simulink model "animation"  (R2018b)
settings: Solver=VariableStepAuto  StartTime=0.0  StopTime=281.0754  FixedStep=0.01  RelTol=1e-3  EnableMultiTasking=on
values from neighbouring files (symbols this model uses):
  cm = [[0.3;49.6;82],[355.2;24;0.7],[9.8;0;36.7],[0.1;246;20],[0;13.9;55],[0;0;59]]    [dynamics.m]    (also in invDynController.m)
  D = generalizedInertiaMatrix(q,rho,DH,m,cm,I)    [dynamics.m]    (also in generalizedInertiaMatrix.m = D + (Si*J(:,:,i))'*Mc_i*(Si*J(:,:,i)); invDynController.m; motionPlanning.m = size(q_new,2); trajGen.m = size(q,1))
  m = [9 4.3 1.9 1.7 0.3 0.1]    [dynamics.m]    (also in invDynController.m)
  N = numel(pos_list)    [missionPlanning.m]    (also in motionPlanning.m = size(q_new,1); simManipulator.m = numel(Path(:,1)); trajGen.m = size(q,2); trajGen_fmincon.m = size(q,2))
undefined symbols (not defined in the file or in its folder): X, Y, Z
libraries: sm_lib x142, nesl_utility x51, simulink x2
(part 2 of 4)

== system animation/Plant/Link5 ==
  Reference Frame4 : sm_lib/Frames and Transforms/Reference Frame
  Revolute Joint4 : sm_lib/Joints/Revolute Joint  SenseConstraintForce=off  SenseConstraintForceX=off  SenseConstraintForceY=off  SenseConstraintForceZ=off  SenseConstraintTorque=off  SenseConstraintTorqueX=off  SenseConstraintTorqueY=off  SenseConstraintTorqueZ=off  SenseTotalForce=off  SenseTotalForceX=off  SenseTotalForceY=off  SenseTotalForceZ=off  SenseTotalTorque=off  SenseTotalTorqueX=off  SenseTotalTorqueY=off  SenseTotalTorqueZ=off  CompositeWrenchDir=FollowerOnBase  CompositeWrenchFrame=BaseFrame  EquilibriumPosition=0  EquilibriumPositionUnits=deg  SpringStiffness=0  SpringStiffnessUnits=N*m/deg  DampingCoefficient=0  DampingCoefficientUnits=N*m/(deg/s)  TorqueActuationMode=InputTorque  MotionActuationMode=ComputedMotion  SensePosition=on  SenseVelocity=on  SenseAcceleration=off  SenseTorqueForce=on  PositionTargetSpecify=on  PositionTargetPriority=High  PositionTargetValue=0  PositionTargetValueUnits=deg  VelocityTargetSpecify=on  VelocityTargetPriority=High  VelocityTargetValue=0  VelocityTargetValueUnits=deg/s
  Rigid Transform13 : sm_lib/Frames and Transforms/Rigid Transform  TranslationMethod=None  TranslationStandardOffset=0  TranslationLengthUnit=m  TranslationStandardAxis=+Z  TranslationCartesianOffset=[0 0 0]  TranslationROffset=0  TranslationROffsetUnits=m  TranslationZOffset=0  TranslationZOffsetUnits=m  TranslationThetaOffset=0  TranslationThetaOffsetUnits=deg  RotationMethod=StandardAxis  RotationAngleUnits=rad  RotationStandardAxis=+Z  RotationAngle=-pi/6  RotationArbitraryAxis=[0 0 1]  FollAlignAxisA=+X  BaseAlignAxisA=+Y  FollAlignAxisB=+Y  BaseAlignAxisB=+Z  RotationSequenceAxes=FollowerAxes  RotationSequence=XYX  RotationSequenceAngles=[0 0 0]  RotationSequenceAnglesUnits=deg  RotationMatrix=[1 0 0; 0 1 0; 0 0 1]
  Rigid Transform14 : sm_lib/Frames and Transforms/Rigid Transform  TranslationMethod=None  TranslationStandardOffset=250.5  TranslationLengthUnit=mm  TranslationStandardAxis=+Z  TranslationCartesianOffset=[0 0 0]  TranslationROffset=0  TranslationROffsetUnits=m  TranslationZOffset=0  TranslationZOffsetUnits=m  TranslationThetaOffset=0  TranslationThetaOffsetUnits=deg  RotationMethod=None  RotationAngleUnits=deg  RotationStandardAxis=+Z  RotationAngle=0.0  RotationArbitraryAxis=[0 0 1]  FollAlignAxisA=+X  BaseAlignAxisA=+Y  FollAlignAxisB=+Y  BaseAlignAxisB=+Z  RotationSequenceAxes=FollowerAxes  RotationSequence=XYX  RotationSequenceAngles=[0 0 0]  RotationSequenceAnglesUnits=deg  RotationMatrix=[1 0 0; 0 1 0; 0 0 1]
  Rigid Transform15 : sm_lib/Frames and Transforms/Rigid Transform  TranslationMethod=None  TranslationStandardOffset=0  TranslationLengthUnit=m  TranslationStandardAxis=+Z  TranslationCartesianOffset=[0 0 0]  TranslationROffset=0  TranslationROffsetUnits=m  TranslationZOffset=0  TranslationZOffsetUnits=m  TranslationThetaOffset=0  TranslationThetaOffsetUnits=deg  RotationMethod=None  RotationAngleUnits=rad  RotationStandardAxis=+X  RotationAngle=pi/2  RotationArbitraryAxis=[0 0 1]  FollAlignAxisA=+X  BaseAlignAxisA=+Y  FollAlignAxisB=+Y  BaseAlignAxisB=+Z  RotationSequenceAxes=FollowerAxes  RotationSequence=XYX  RotationSequenceAngles=[0 0 0]  RotationSequenceAnglesUnits=deg  RotationMatrix=[1 0 0; 0 1 0; 0 0 1]
  Rigid Transform20 : sm_lib/Frames and Transforms/Rigid Transform  TranslationMethod=None  TranslationStandardOffset=500  TranslationLengthUnit=mm  TranslationStandardAxis=+X  TranslationCartesianOffset=[0 0 0]  TranslationROffset=0  TranslationROffsetUnits=m  TranslationZOffset=0  TranslationZOffsetUnits=m  TranslationThetaOffset=0  TranslationThetaOffsetUnits=deg  RotationMethod=StandardAxis  RotationAngleUnits=rad  RotationStandardAxis=+X  RotationAngle=-pi/2  RotationArbitraryAxis=[0 0 1]  FollAlignAxisA=+X  BaseAlignAxisA=+Y  FollAlignAxisB=+Y  BaseAlignAxisB=+Z  RotationSequenceAxes=FollowerAxes  RotationSequence=XYX  RotationSequenceAngles=[0 0 0]  RotationSequenceAnglesUnits=deg  RotationMatrix=[1 0 0; 0 1 0; 0 0 1]
  Solid5 : sm_lib/Body Elements/Solid  InertiaType=Custom  Mass=0.87  MassUnits=kg  CenterOfMass=[0 4.29 -58.96]  CenterOfMassUnits=mm  MomentsOfInertia=[0 0 0]  MomentsOfInertiaUnits=kg*m^2  ProductsOfInertia=[0 0 0]  ProductsOfInertiaUnits=kg*m^2  BasedOnType=Density  Density=1000  DensityUnits=kg/m^3  DoExposeReferenceFrame=on  SerializedFrames=<Frames/>  GraphicType=FromGeometry  MarkerShape=Sphere  MarkerSize=10  GraphicVisPropType=SimpleVisualProperties  GraphicDiffuseColor=[1.0 1.0 0.0]  GraphicSpecularColor=[0.5 0.5 0.5 1.0]  GraphicAmbientColor=[0.15 0.15 0.15 1.0]  GraphicEmissiveColor=[0.0 0.0 0.0 1.0]  GraphicShininess=75  GraphicOpacity=1.0  GeometryShape=FromFile  RectangleSize=[1 1]  RectangleSizeUnits=m  BrickDimensions=[1 1 1]  BrickDimensionUnits=m  CylinderRadius=1  CylinderRadiusUnits=m  CylinderLength=1  CylinderLengthUnits=m  SphereRadius=1  SphereRadiusUnits=m  EllipsoidRadii=[1 1 1]  EllipsoidRadiiUnits=m  ExtrusionCrossSection=[1 1; -1 1; -1 -1; 1 -1]  ExtrusionCrossSectionUnits=m  ExtrusionLength=1  ExtrusionLengthUnits=m  PolygonNumSides=3  PolygonOuterRadius=1  PolygonOuterRadiusUnits=m  ExtGeomFileType=STL  ExtGeomFileName=D:\Chin\3rdYearsProject\IntroRobotics\Project\CAD\SubAssem6.STL  ExtGeomFileUnits=mm  RevolutionCrossSection=[1 1; 1 -1; 2 -1; 2 1]  RevolutionCrossSectionUnits=m  RevolutionExtent=Full  RevolutionAngle=180  RevolutionAngleUnits=deg
  Frame4 : PMIOPort  Side=Left
  t : PMIOPort  Port=2  Side=Left
  Frame5 : PMIOPort  Port=3  Side=Right
  q : PMIOPort  Port=4  Side=Right
  w : PMIOPort  Port=5  Side=Right
  t_out : PMIOPort  Port=6  Side=Right
  connections:
  Rigid Transform20/RConn1 -- Frame5/RConn1 -- Reference Frame4/RConn1 -- Solid5/RConn1
  Rigid Transform15/LConn1 -- Rigid Transform14/RConn1
  Rigid Transform15/RConn1 -- Rigid Transform20/LConn1
  Rigid Transform13/LConn1 -- Revolute Joint4/RConn1
  Rigid Transform14/LConn1 -- Rigid Transform13/RConn1
  Revolute Joint4/LConn1 -- Frame4/RConn1
  Revolute Joint4/LConn2 -- t/RConn1
  Revolute Joint4/RConn3 -- w/RConn1
  Revolute Joint4/RConn2 -- q/RConn1
  Revolute Joint4/RConn4 -- t_out/RConn1

== system animation/Plant/Link6 ==
  Reference Frame5 : sm_lib/Frames and Transforms/Reference Frame
  Revolute Joint5 : sm_lib/Joints/Revolute Joint  SenseConstraintForce=off  SenseConstraintForceX=off  SenseConstraintForceY=off  SenseConstraintForceZ=off  SenseConstraintTorque=off  SenseConstraintTorqueX=off  SenseConstraintTorqueY=off  SenseConstraintTorqueZ=off  SenseTotalForce=off  SenseTotalForceX=off  SenseTotalForceY=off  SenseTotalForceZ=off  SenseTotalTorque=off  SenseTotalTorqueX=off  SenseTotalTorqueY=off  SenseTotalTorqueZ=off  CompositeWrenchDir=FollowerOnBase  CompositeWrenchFrame=BaseFrame  EquilibriumPosition=0  EquilibriumPositionUnits=deg  SpringStiffness=0  SpringStiffnessUnits=N*m/deg  DampingCoefficient=0  DampingCoefficientUnits=N*m/(deg/s)  TorqueActuationMode=InputTorque  MotionActuationMode=ComputedMotion  SensePosition=on  SenseVelocity=on  SenseAcceleration=off  SenseTorqueForce=on  PositionTargetSpecify=on  PositionTargetPriority=High  PositionTargetValue=0  PositionTargetValueUnits=deg  VelocityTargetSpecify=on  VelocityTargetPriority=High  VelocityTargetValue=0  VelocityTargetValueUnits=deg/s
  Rigid Transform21 : sm_lib/Frames and Transforms/Rigid Transform  TranslationMethod=None  TranslationStandardOffset=0  TranslationLengthUnit=m  TranslationStandardAxis=+Z  TranslationCartesianOffset=[0 0 0]  TranslationROffset=0  TranslationROffsetUnits=m  TranslationZOffset=0  TranslationZOffsetUnits=m  TranslationThetaOffset=0  TranslationThetaOffsetUnits=deg  RotationMethod=None  RotationAngleUnits=rad  RotationStandardAxis=+Z  RotationAngle=-pi/6  RotationArbitraryAxis=[0 0 1]  FollAlignAxisA=+X  BaseAlignAxisA=+Y  FollAlignAxisB=+Y  BaseAlignAxisB=+Z  RotationSequenceAxes=FollowerAxes  RotationSequence=XYX  RotationSequenceAngles=[0 0 0]  RotationSequenceAnglesUnits=deg  RotationMatrix=[1 0 0; 0 1 0; 0 0 1]
  Rigid Transform22 : sm_lib/Frames and Transforms/Rigid Transform  TranslationMethod=StandardAxis  TranslationStandardOffset=230  TranslationLengthUnit=mm  TranslationStandardAxis=-Z  TranslationCartesianOffset=[0 0 0]  TranslationROffset=0  TranslationROffsetUnits=m  TranslationZOffset=0  TranslationZOffsetUnits=m  TranslationThetaOffset=0  TranslationThetaOffsetUnits=deg  RotationMethod=None  RotationAngleUnits=deg  RotationStandardAxis=+Z  RotationAngle=0.0  RotationArbitraryAxis=[0 0 1]  FollAlignAxisA=+X  BaseAlignAxisA=+Y  FollAlignAxisB=+Y  BaseAlignAxisB=+Z  RotationSequenceAxes=FollowerAxes  RotationSequence=XYX  RotationSequenceAngles=[0 0 0]  RotationSequenceAnglesUnits=deg  RotationMatrix=[1 0 0; 0 1 0; 0 0 1]
  Rigid Transform23 : sm_lib/Frames and Transforms/Rigid Transform  TranslationMethod=None  TranslationStandardOffset=0  TranslationLengthUnit=m  TranslationStandardAxis=+Z  TranslationCartesianOffset=[0 0 0]  TranslationROffset=0  TranslationROffsetUnits=m  TranslationZOffset=0  TranslationZOffsetUnits=m  TranslationThetaOffset=0  TranslationThetaOffsetUnits=deg  RotationMethod=None  RotationAngleUnits=rad  RotationStandardAxis=+X  RotationAngle=pi/2  RotationArbitraryAxis=[0 0 1]  FollAlignAxisA=+X  BaseAlignAxisA=+Y  FollAlignAxisB=+Y  BaseAlignAxisB=+Z  RotationSequenceAxes=FollowerAxes  RotationSequence=XYX  RotationSequenceAngles=[0 0 0]  RotationSequenceAnglesUnits=deg  RotationMatrix=[1 0 0; 0 1 0; 0 0 1]
  Rigid Transform24 : sm_lib/Frames and Transforms/Rigid Transform  TranslationMethod=None  TranslationStandardOffset=500  TranslationLengthUnit=mm  TranslationStandardAxis=+X  TranslationCartesianOffset=[0 0 0]  TranslationROffset=0  TranslationROffsetUnits=m  TranslationZOffset=0  TranslationZOffsetUnits=m  TranslationThetaOffset=0  TranslationThetaOffsetUnits=deg  RotationMethod=StandardAxis  RotationAngleUnits=rad  RotationStandardAxis=+X  RotationAngle=pi  RotationArbitraryAxis=[0 0 1]  FollAlignAxisA=+X  BaseAlignAxisA=+Y  FollAlignAxisB=+Y  BaseAlignAxisB=+Z  RotationSequenceAxes=FollowerAxes  RotationSequence=XYX  RotationSequenceAngles=[0 0 0]  RotationSequenceAnglesUnits=deg  RotationMatrix=[1 0 0; 0 1 0; 0 0 1]
  Solid6 : sm_lib/Body Elements/Solid  InertiaType=Custom  Mass=0.115  MassUnits=kg  CenterOfMass=[-1.12 -0.51 -58.13]  CenterOfMassUnits=mm  MomentsOfInertia=[5029.75 5041.84 923.6]  MomentsOfInertiaUnits=g*cm^2  ProductsOfInertia=[39.56 88.09 6.8]  ProductsOfInertiaUnits=g*cm^2  BasedOnType=Density  Density=1000  DensityUnits=kg/m^3  DoExposeReferenceFrame=on  SerializedFrames=<Frames/>  GraphicType=FromGeometry  MarkerShape=Sphere  MarkerSize=10  GraphicVisPropType=SimpleVisualProperties  GraphicDiffuseColor=[0.0 1.0 0.2]  GraphicSpecularColor=[0.5 0.5 0.5 1.0]  GraphicAmbientColor=[0.15 0.15 0.15 1.0]  GraphicEmissiveColor=[0.0 0.0 0.0 1.0]  GraphicShininess=75  GraphicOpacity=1.0  GeometryShape=FromFile  RectangleSize=[1 1]  RectangleSizeUnits=m  BrickDimensions=[1 1 1]  BrickDimensionUnits=m  CylinderRadius=1  CylinderRadiusUnits=m  CylinderLength=1  CylinderLengthUnits=m  SphereRadius=1  SphereRadiusUnits=m  EllipsoidRadii=[1 1 1]  EllipsoidRadiiUnits=m  ExtrusionCrossSection=[1 1; -1 1; -1 -1; 1 -1]  ExtrusionCrossSectionUnits=m  ExtrusionLength=1  ExtrusionLengthUnits=m  PolygonNumSides=3  PolygonOuterRadius=1  PolygonOuterRadiusUnits=m  ExtGeomFileType=STL  ExtGeomFileName=D:\Chin\3rdYearsProject\IntroRobotics\Project\CAD\SubAssem_end_plate2.STL  ExtGeomFileUnits=mm  RevolutionCrossSection=[1 1; 1 -1; 2 -1; 2 1]  RevolutionCrossSectionUnits=m  RevolutionExtent=Full  RevolutionAngle=180  RevolutionAngleUnits=deg
  Frame6 : PMIOPort  Side=Left
  Frame5 : PMIOPort  Port=2  Side=Right
  t : PMIOPort  Port=3  Side=Left
  q : PMIOPort  Port=4  Side=Right
  w : PMIOPort  Port=5  Side=Right
  t_out : PMIOPort  Port=6  Side=Right
  connections:
  Revolute Joint5/LConn2 -- t/RConn1
  Revolute Joint5/RConn3 -- w/RConn1
  Revolute Joint5/RConn2 -- q/RConn1
  Rigid Transform24/RConn1 -- Solid6/RConn1 -- Frame6/RConn1 -- Reference Frame5/RConn1
  Rigid Transform22/LConn1 -- Rigid Transform21/RConn1
  Rigid Transform23/RConn1 -- Rigid Transform24/LConn1
  Rigid Transform23/LConn1 -- Rigid Transform22/RConn1
  Rigid Transform21/LConn1 -- Revolute Joint5/RConn1
  Revolute Joint5/LConn1 -- Frame5/RConn1
  t_out/RConn1 -- Revolute Joint5/RConn4

== system animation/Trajectory Generator/Trajectory1 ==
  t : Inport
  A : Subsystem
  Product : Product  Multiplication=Matrix(*)
  Product1 : Product  Multiplication=Matrix(*)
  Product2 : Product  Multiplication=Matrix(*)
  coef_q : Subsystem
  coef_qd : Subsystem
  coef_qdd : Subsystem
  q_r : Outport
  qd_r : Outport  Port=2
  qdd_r : Outport  Port=3
  wires:
  Product/1 -> q_r/1
  A/1(A) -> Product2/2, Product1/2, Product/2
  coef_qd/1(coef_qd) -> Product1/1
  coef_qdd/1(coef_qdd) -> Product2/1
  t/1 -> coef_qdd/1(t), coef_qd/1(t), coef_q/1(t)
  Product1/1 -> qd_r/1
  coef_q/1(coef_q) -> Product/1
  Product2/1 -> qdd_r/1

== system animation/Trajectory Generator/Trajectory2 ==
  t : Inport
  A : Subsystem
  Product : Product  Multiplication=Matrix(*)
  Product1 : Product  Multiplication=Matrix(*)
  Product2 : Product  Multiplication=Matrix(*)
  coef_q : Subsystem
  coef_qd : Subsystem
  coef_qdd : Subsystem
  q_r : Outport
  qd_r : Outport  Port=2
  qdd_r : Outport  Port=3
  wires:
  Product2/1 -> qdd_r/1
  coef_q/1(coef_q) -> Product/1
  Product1/1 -> qd_r/1
  t/1 -> coef_q/1(t), coef_qd/1(t), coef_qdd/1(t)
  coef_qdd/1(coef_qdd) -> Product2/1
  coef_qd/1(coef_qd) -> Product1/1
  A/1(A) -> Product/2, Product1/2, Product2/2
  Product/1 -> q_r/1

== system animation/Trajectory Generator/Trajectory3 ==
  t : Inport
  A : Subsystem
  Product : Product  Multiplication=Matrix(*)
  Product1 : Product  Multiplication=Matrix(*)
  Product2 : Product  Multiplication=Matrix(*)
  coef_q : Subsystem
  coef_qd : Subsystem
  coef_qdd : Subsystem
  q_r : Outport
  qd_r : Outport  Port=2
  qdd_r : Outport  Port=3
  wires:
  Product/1 -> q_r/1
  A/1(A) -> Product2/2, Product1/2, Product/2
  coef_qd/1(coef_qd) -> Product1/1
  coef_qdd/1(coef_qdd) -> Product2/1
  t/1 -> coef_qdd/1(t), coef_qd/1(t), coef_q/1(t)
  Product1/1 -> qd_r/1
  coef_q/1(coef_q) -> Product/1
  Product2/1 -> qdd_r/1

== system animation/Trajectory Generator1/Trajectory2 ==
  t : Inport
  A : Subsystem
  Product : Product  Multiplication=Matrix(*)
  Product1 : Product  Multiplication=Matrix(*)
  Product2 : Product  Multiplication=Matrix(*)
  coef_q : Subsystem
  coef_qd : Subsystem
  coef_qdd : Subsystem
  q_r : Outport
  qd_r : Outport  Port=2
  qdd_r : Outport  Port=3
  wires:
  Product/1 -> q_r/1
  A/1(A) -> Product2/2, Product1/2, Product/2
  coef_qd/1(coef_qd) -> Product1/1
  coef_qdd/1(coef_qdd) -> Product2/1
  t/1 -> coef_qdd/1(t), coef_qd/1(t), coef_q/1(t)
  Product1/1 -> qd_r/1
  coef_q/1(coef_q) -> Product/1
  Product2/1 -> qdd_r/1

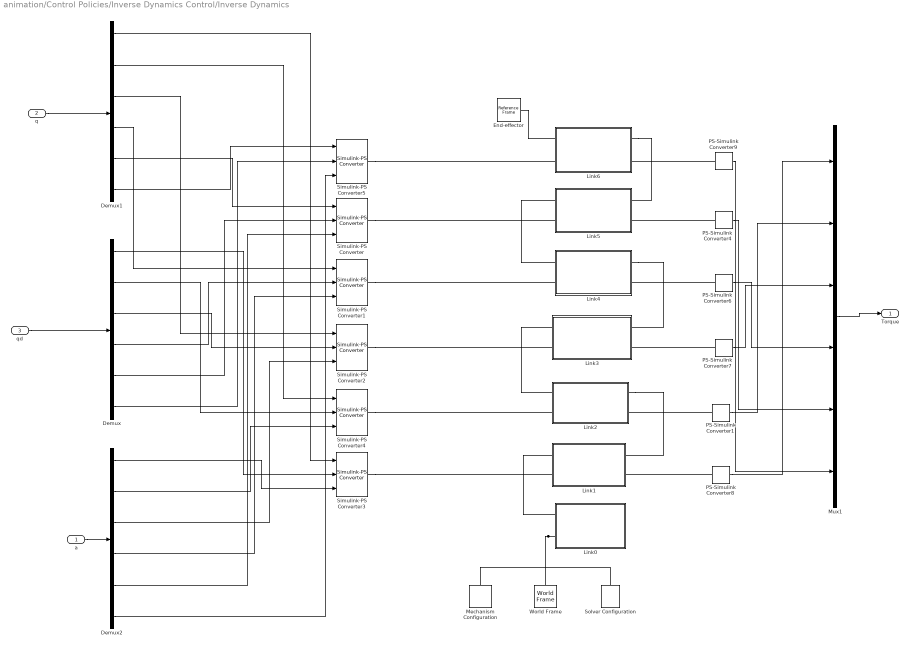
== system animation/Control Policies/Inverse Dynamics Control/Inverse Dynamics ==
  a : Inport
  q : Inport  Port=2
  qd : Inport  Port=3
  Demux : Demux  Outputs=6
  Demux1 : Demux  Outputs=6
  Demux2 : Demux  Outputs=6
  End-effector : sm_lib/Frames and Transforms/Reference Frame
  Link0 : Subsystem
  Link1 : Subsystem
  Link2 : Subsystem
  Link3 : Subsystem
  Link4 : Subsystem
  Link5 : Subsystem
  Link6 : Subsystem
  Mechanism Configuration : sm_lib/Utilities/Mechanism Configuration  UniformGravity=Constant  GravityVector=[0 0 -9.80665]  GravityUnits=m/s^2  LinearizationDelta=0.001
  Mux1 : Mux  Inputs=6
  PS-Simulink Converter{1,4,6..9} (6 alike) : nesl_utility/PS-Simulink Converter  PhysicalDomain=network_engine_domain  SubClassName=ps_output  LeftPortType=input  RightPortType=output  PseudoPeriodic=off  Frequencies=[]  Unit=1  AffineConversion=off
  Simulink-PS Converter{,1..5} (6 alike) : nesl_utility/Simulink-PS Converter  PhysicalDomain=network_engine_domain  SubClassName=ps_input  LeftPortType=input  RightPortType=output  PseudoPeriodic=off  Frequencies=[]  NoiseDistribution=none  NoiseParameters=[]  Unit=1  AffineConversion=off  FilteringAndDerivatives=provide  SimscapeFilterOrder=1  InputFilterTimeConstant=0.001  UdotUserProvided=2
  Solver Configuration : nesl_utility/Solver Configuration  PhysicalDomain=network_engine_domain  SubClassName=solver  LeftPortType=input  RightPortType=generic  Tones=[]  Harmonics=[]  SimulateNoise=off  Profile=off  UseLocalSampling=off  EnableSwitchedLinearOptims=on  FrequencyDomain=off  UseCCode=off  RelTol=0.001  AbsTol=1e-06  MinStep=1e-09  ToWorkspace=off  RevertToSquareIcSolve=off  NumHomotopyIterations=100  PhasorMode=off  PhasorModeNumHarmonics=1  DoDC=off  ResidualTolerance=1e-09  UseLocalSolver=off  LocalSolverChoice=NE_BACKWARD_EULER_ADVANCER  LocalSolverSampleTime=0.001  DoFixedCost=off  MaxNonlinIter=3  MaxModeIter=2  LinearAlgebra=Sparse  EquationFormulation=NE_TIME_EF  DelaysMemoryBudget=1024  AutomaticFiltering=on  FilteringTimeConstant=0.001  PartitionStorageMethod=AS_NEEDED  PartitionMemoryBudget=1024
  World Frame : sm_lib/Frames and Transforms/World Frame
  "Torque " : Outport
  wires:
  Mux1/1 -> "Torque "/1
  q/1 -> Demux1/1
  a/1 -> Demux2/1
  qd/1 -> Demux/1
  Demux1/6 -> Simulink-PS Converter5/1
  Demux1/5 -> Simulink-PS Converter/1
  Demux1/4 -> Simulink-PS Converter1/1
  Demux1/3 -> Simulink-PS Converter2/1
  Demux1/2 -> Simulink-PS Converter4/1
  Demux1/1 -> Simulink-PS Converter3/1
  Demux/1 -> Simulink-PS Converter3/2
  Demux/2 -> Simulink-PS Converter4/2
  Demux/3 -> Simulink-PS Converter2/2
  Demux/4 -> Simulink-PS Converter1/2
  Demux/5 -> Simulink-PS Converter/2
  Demux/6 -> Simulink-PS Converter5/2
  Demux2/1 -> Simulink-PS Converter3/3
  Demux2/2 -> Simulink-PS Converter4/3
  Demux2/3 -> Simulink-PS Converter2/3
  Demux2/4 -> Simulink-PS Converter1/3
  Demux2/5 -> Simulink-PS Converter/3
  Demux2/6 -> Simulink-PS Converter5/3
  PS-Simulink Converter8/1 -> Mux1/1
  PS-Simulink Converter1/1 -> Mux1/2
  PS-Simulink Converter7/1 -> Mux1/3
  PS-Simulink Converter6/1 -> Mux1/4
  PS-Simulink Converter4/1 -> Mux1/5
  PS-Simulink Converter9/1 -> Mux1/6
  connections:
  End-effector/RConn1 -- Link6/LConn1
  Link3/LConn1 -- Link2/LConn1
  Link6/RConn1 -- Link5/RConn1
  Link5/LConn1 -- Link4/LConn1
  Link4/RConn1 -- Link3/RConn1
  Link1/LConn1 -- Link0/LConn1
  Link2/RConn1 -- Link1/RConn1
  Link0/LConn2 -- Mechanism Configuration/RConn1 -- World Frame/RConn1 -- Solver Configuration/RConn1
  Simulink-PS Converter/RConn1 -- Link5/LConn2
  Simulink-PS Converter1/RConn1 -- Link4/LConn2
  Simulink-PS Converter2/RConn1 -- Link3/LConn2
  Simulink-PS Converter4/RConn1 -- Link2/LConn2
  Simulink-PS Converter3/RConn1 -- Link1/LConn2
  Simulink-PS Converter5/RConn1 -- Link6/LConn2
  PS-Simulink Converter4/LConn1 -- Link5/RConn2
  PS-Simulink Converter6/LConn1 -- Link4/RConn2
  PS-Simulink Converter9/LConn1 -- Link6/RConn2
  PS-Simulink Converter7/LConn1 -- Link3/RConn2
  PS-Simulink Converter1/LConn1 -- Link2/RConn2
  PS-Simulink Converter8/LConn1 -- Link1/RConn2

== system animation/Control Policies/Inverse Dynamics Control/Outer_loop ==
  q_r : Inport
  qd_r : Inport  Port=2
  qdd_r : Inport  Port=3
  q : Inport  Port=4
  qd : Inport  Port=5
  Gain : Gain  Gain=Kp1  Multiplication=Matrix(K*u)
  Gain1 : Gain  Gain=Kd1  Multiplication=Matrix(K*u)
  Sum : Sum  Inputs=|++
  Sum1 : Sum  Inputs=|++
  Sum2 : Sum  Inputs=|+-
  Sum3 : Sum  Inputs=|+-
  a : Outport
  wires:
  qdd_r/1 -> Sum/1
  Sum3/1 -> Gain1/1  "eqd"
  Sum2/1 -> Gain/1  "eq"
  q_r/1 -> Sum2/1
  Sum/1 -> a/1
  qd_r/1 -> Sum3/1
  qd/1 -> Sum3/2
  q/1 -> Sum2/2
  Gain/1 -> Sum1/1
  Sum1/1 -> Sum/2
  Gain1/1 -> Sum1/2

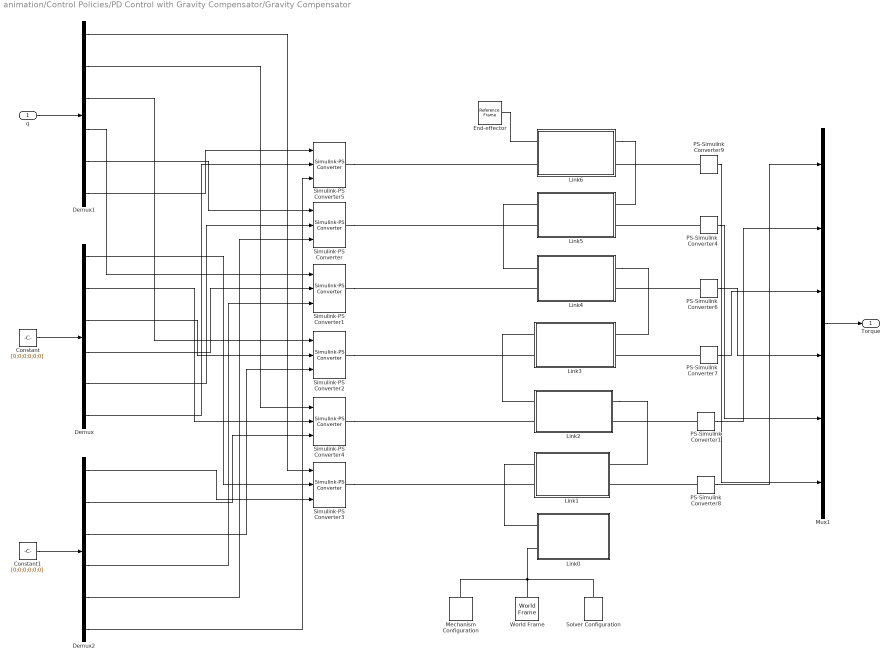
== system animation/Control Policies/PD Control with Gravity Compensator/Gravity Compensator ==
  q : Inport
  Constant : Constant  Value=[0;0;0;0;0;0]
  Constant1 : Constant  Value=[0;0;0;0;0;0]
  Demux : Demux  Outputs=6
  Demux1 : Demux  Outputs=6
  Demux2 : Demux  Outputs=6
  End-effector : sm_lib/Frames and Transforms/Reference Frame
  Link0 : Subsystem
  Link1 : Subsystem
  Link2 : Subsystem
  Link3 : Subsystem
  Link4 : Subsystem
  Link5 : Subsystem
  Link6 : Subsystem
  Mechanism Configuration : sm_lib/Utilities/Mechanism Configuration  UniformGravity=Constant  GravityVector=[0 0 -9.80665]  GravityUnits=m/s^2  LinearizationDelta=0.001
  Mux1 : Mux  Inputs=6
  PS-Simulink Converter{1,4,6..9} (6 alike) : nesl_utility/PS-Simulink Converter  PhysicalDomain=network_engine_domain  SubClassName=ps_output  LeftPortType=input  RightPortType=output  PseudoPeriodic=off  Frequencies=[]  Unit=1  AffineConversion=off
  Simulink-PS Converter{,1..5} (6 alike) : nesl_utility/Simulink-PS Converter  PhysicalDomain=network_engine_domain  SubClassName=ps_input  LeftPortType=input  RightPortType=output  PseudoPeriodic=off  Frequencies=[]  NoiseDistribution=none  NoiseParameters=[]  Unit=1  AffineConversion=off  FilteringAndDerivatives=provide  SimscapeFilterOrder=1  InputFilterTimeConstant=0.001  UdotUserProvided=2
  Solver Configuration : nesl_utility/Solver Configuration  PhysicalDomain=network_engine_domain  SubClassName=solver  LeftPortType=input  RightPortType=generic  Tones=[]  Harmonics=[]  SimulateNoise=off  Profile=off  UseLocalSampling=off  EnableSwitchedLinearOptims=on  FrequencyDomain=off  UseCCode=off  RelTol=0.001  AbsTol=1e-06  MinStep=1e-09  ToWorkspace=off  RevertToSquareIcSolve=off  NumHomotopyIterations=100  PhasorMode=off  PhasorModeNumHarmonics=1  DoDC=off  ResidualTolerance=1e-09  UseLocalSolver=off  LocalSolverChoice=NE_BACKWARD_EULER_ADVANCER  LocalSolverSampleTime=0.001  DoFixedCost=off  MaxNonlinIter=3  MaxModeIter=2  LinearAlgebra=Sparse  EquationFormulation=NE_TIME_EF  DelaysMemoryBudget=1024  AutomaticFiltering=on  FilteringTimeConstant=0.001  PartitionStorageMethod=AS_NEEDED  PartitionMemoryBudget=1024
  World Frame : sm_lib/Frames and Transforms/World Frame
  "Torque " : Outport
  wires:
  PS-Simulink Converter9/1 -> Mux1/6
  PS-Simulink Converter4/1 -> Mux1/5
  PS-Simulink Converter6/1 -> Mux1/4
  PS-Simulink Converter7/1 -> Mux1/3
  PS-Simulink Converter1/1 -> Mux1/2
  PS-Simulink Converter8/1 -> Mux1/1
  Demux2/6 -> Simulink-PS Converter5/3
  Demux2/5 -> Simulink-PS Converter/3
  Demux2/4 -> Simulink-PS Converter1/3
  Demux2/3 -> Simulink-PS Converter2/3
  Demux2/2 -> Simulink-PS Converter4/3
  Demux2/1 -> Simulink-PS Converter3/3
  Demux/6 -> Simulink-PS Converter5/2
  Demux/5 -> Simulink-PS Converter/2
  Demux/4 -> Simulink-PS Converter1/2
  Demux/3 -> Simulink-PS Converter2/2
  Demux/2 -> Simulink-PS Converter4/2
  Demux/1 -> Simulink-PS Converter3/2
  Demux1/1 -> Simulink-PS Converter3/1
  Demux1/2 -> Simulink-PS Converter4/1
  Demux1/3 -> Simulink-PS Converter2/1
  Demux1/4 -> Simulink-PS Converter1/1
  Demux1/5 -> Simulink-PS Converter/1
  Demux1/6 -> Simulink-PS Converter5/1
  Constant/1 -> Demux/1
  Constant1/1 -> Demux2/1
  q/1 -> Demux1/1
  Mux1/1 -> "Torque "/1
  connections:
  PS-Simulink Converter8/LConn1 -- Link1/RConn2
  PS-Simulink Converter1/LConn1 -- Link2/RConn2
  PS-Simulink Converter7/LConn1 -- Link3/RConn2
  PS-Simulink Converter9/LConn1 -- Link6/RConn2
  PS-Simulink Converter6/LConn1 -- Link4/RConn2
  PS-Simulink Converter4/LConn1 -- Link5/RConn2
  Simulink-PS Converter5/RConn1 -- Link6/LConn2
  Simulink-PS Converter3/RConn1 -- Link1/LConn2
  Simulink-PS Converter4/RConn1 -- Link2/LConn2
  Simulink-PS Converter2/RConn1 -- Link3/LConn2
  Simulink-PS Converter1/RConn1 -- Link4/LConn2
  Simulink-PS Converter/RConn1 -- Link5/LConn2
  Solver Configuration/RConn1 -- World Frame/RConn1 -- Mechanism Configuration/RConn1 -- Link0/LConn2
  Link2/RConn1 -- Link1/RConn1
  Link1/LConn1 -- Link0/LConn1
  Link4/RConn1 -- Link3/RConn1
  Link5/LConn1 -- Link4/LConn1
  Link6/RConn1 -- Link5/RConn1
  Link3/LConn1 -- Link2/LConn1
  End-effector/RConn1 -- Link6/LConn1

== system animation/Control Policies/PD Control with Gravity Compensator/PD control ==
  compensate : Inport
  q_r : Inport  Port=2
  qd_r : Inport  Port=3
  q : Inport  Port=4
  qd : Inport  Port=5
  Gain : Gain  Gain=Kp2  Multiplication=Matrix(K*u)
  Gain1 : Gain  Gain=Kd2  Multiplication=Matrix(K*u)
  Sum : Sum  Inputs=|+-
  Sum1 : Sum  Inputs=|+-
  Sum2 : Sum  Inputs=+|+|+
  u : Outport
  wires:
  Gain1/1 -> Sum2/3
  q_r/1 -> Sum/1
  Sum2/1 -> u/1
  Sum1/1 -> Gain1/1
  qd_r/1 -> Sum1/1
  Gain/1 -> Sum2/2
  Sum/1 -> Gain/1
  q/1 -> Sum/2
  qd/1 -> Sum1/2
  compensate/1 -> Sum2/1

== system animation/Trajectory Generator/Trajectory1/A ==
  Constant : Constant  Value=[eye(6) zeros(6) zeros(6) zeros(6) zeros(6) zeros(6)]
  Constant1 : Constant  Value=[eye(6) eye(6)*T eye(6)*T^2 eye(6)*T^3 eye(6)*T^4 eye(6)*T^5]
  Constant2 : Constant  Value=[zeros(6) eye(6) zeros(6) zeros(6) zeros(6) zeros(6)]
  Constant3 : Constant  Value=[zeros(6) eye(6) eye(6)*2*T eye(6)*3*T^2 eye(6)*4*T^3 eye(6)*5*T^4]
  Constant4 : Constant  Value=[zeros(6) zeros(6) 2*eye(6) zeros(6) zeros(6) zeros(6)]
  Constant5 : Constant  Value=[zeros(6) zeros(6) 2*eye(6) 6*T*eye(6) 12*T^2*eye(6) 20*T^3*eye(6)]
  Divide : Product  Inputs=/  Multiplication=Matrix(*)
  Matrix Concatenate : Concatenate  NumInputs=6  Mode=Multidimensional array
  Matrix Concatenate1 : Concatenate  NumInputs=6  Mode=Multidimensional array
  O{,1..4} (5 alike) : Constant  Value=zeros(6,1)
  Product : Product  Multiplication=Matrix(*)
  q_T : Constant  Value=q1
  A : Outport
  wires:
  O3/1 -> Matrix Concatenate/5
  O/1 -> Matrix Concatenate/1
  q_T/1 -> Matrix Concatenate/2
  O4/1 -> Matrix Concatenate/6
  O2/1 -> Matrix Concatenate/4
  O1/1 -> Matrix Concatenate/3
  Constant/1 -> Matrix Concatenate1/1
  Constant1/1 -> Matrix Concatenate1/2
  Constant2/1 -> Matrix Concatenate1/3
  Constant3/1 -> Matrix Concatenate1/4
  Constant4/1 -> Matrix Concatenate1/5
  Constant5/1 -> Matrix Concatenate1/6
  Matrix Concatenate1/1 -> Divide/1
  Matrix Concatenate/1 -> Product/2
  Divide/1 -> Product/1
  Product/1 -> A/1

== system animation/Trajectory Generator/Trajectory1/coef_q ==
  t : Inport
  Constant1 : Constant  Value=2
  Constant2 : Constant  Value=3
  Constant3 : Constant  Value=4
  Constant4 : Constant  Value=5
  Divide{,1..4} (5 alike) : Product  Inputs=**
  I : Constant  Value=eye(6)
  Math Function{1..4} (4 alike) : Math  Operator=pow  SaturateOnIntegerOverflow=on
  Matrix Concatenate : Concatenate  NumInputs=6  Mode=Multidimensional array  ConcatenateDimension=2
  coef_q : Outport
  wires:
  Divide/1 -> Matrix Concatenate/2
  Matrix Concatenate/1 -> coef_q/1
  I/1 -> Matrix Concatenate/1, Divide4/2, Divide3/2, Divide2/2, Divide1/2, Divide/2
  Constant1/1 -> Math Function1/2
  Divide3/1 -> Matrix Concatenate/5
  Divide1/1 -> Matrix Concatenate/3
  Math Function4/1 -> Divide4/1
  Constant3/1 -> Math Function3/2
  Divide2/1 -> Matrix Concatenate/4
  Constant4/1 -> Math Function4/2
  Math Function3/1 -> Divide3/1
  t/1 -> Divide/1, Math Function3/1, Math Function4/1, Math Function2/1, Math Function1/1
  Math Function1/1 -> Divide1/1
  Constant2/1 -> Math Function2/2
  Math Function2/1 -> Divide2/1
  Divide4/1 -> Matrix Concatenate/6

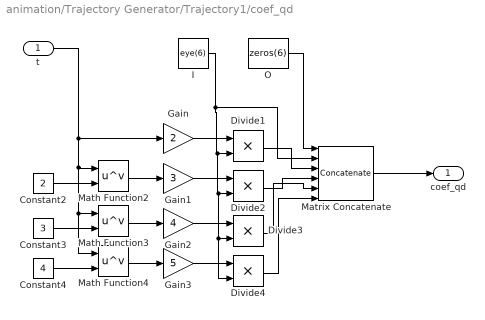
== system animation/Trajectory Generator/Trajectory1/coef_qd ==
  t : Inport
  Constant2 : Constant  Value=2
  Constant3 : Constant  Value=3
  Constant4 : Constant  Value=4
  Divide{1..4} (4 alike) : Product  Inputs=**
  Gain : Gain  Gain=2
  Gain1 : Gain  Gain=3
  Gain2 : Gain  Gain=4
  Gain3 : Gain  Gain=5
  I : Constant  Value=eye(6)
  Math Function2 : Math  Operator=pow  SaturateOnIntegerOverflow=on
  Math Function3 : Math  Operator=pow  SaturateOnIntegerOverflow=on
  Math Function4 : Math  Operator=pow  SaturateOnIntegerOverflow=on
  Matrix Concatenate : Concatenate  NumInputs=6  Mode=Multidimensional array  ConcatenateDimension=2
  O : Constant  Value=zeros(6)
  coef_qd : Outport
  wires:
  Divide4/1 -> Matrix Concatenate/6
  Math Function2/1 -> Gain1/1
  Constant2/1 -> Math Function2/2
  t/1 -> Gain/1, Math Function2/1, Math Function4/1, Math Function3/1
  Math Function3/1 -> Gain2/1
  Constant4/1 -> Math Function4/2
  Divide2/1 -> Matrix Concatenate/4
  Constant3/1 -> Math Function3/2
  Math Function4/1 -> Gain3/1
  Divide1/1 -> Matrix Concatenate/3
  Divide3/1 -> Matrix Concatenate/5
  Matrix Concatenate/1 -> coef_qd/1
  I/1 -> Matrix Concatenate/2, Divide1/2, Divide2/2, Divide3/2, Divide4/2
  O/1 -> Matrix Concatenate/1
  Gain/1 -> Divide1/1
  Gain1/1 -> Divide2/1
  Gain2/1 -> Divide3/1
  Gain3/1 -> Divide4/1

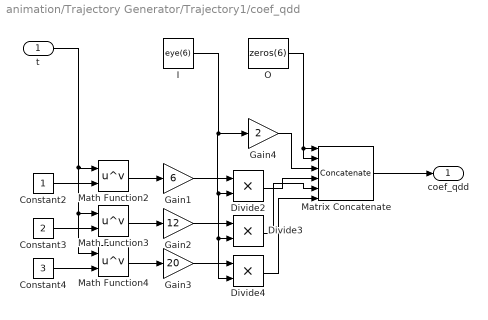
== system animation/Trajectory Generator/Trajectory1/coef_qdd ==
  t : Inport
  Constant2 : Constant
  Constant3 : Constant  Value=2
  Constant4 : Constant  Value=3
  Divide2 : Product  Inputs=**
  Divide3 : Product  Inputs=**
  Divide4 : Product  Inputs=**
  Gain1 : Gain  Gain=6
  Gain2 : Gain  Gain=12
  Gain3 : Gain  Gain=20
  Gain4 : Gain  Gain=2
  I : Constant  Value=eye(6)
  Math Function2 : Math  Operator=pow  SaturateOnIntegerOverflow=on
  Math Function3 : Math  Operator=pow  SaturateOnIntegerOverflow=on
  Math Function4 : Math  Operator=pow  SaturateOnIntegerOverflow=on
  Matrix Concatenate : Concatenate  NumInputs=6  Mode=Multidimensional array  ConcatenateDimension=2
  O : Constant  Value=zeros(6)
  coef_qdd : Outport
  wires:
  Gain3/1 -> Divide4/1
  Gain2/1 -> Divide3/1
  Gain1/1 -> Divide2/1
  O/1 -> Matrix Concatenate/2, Matrix Concatenate/1
  I/1 -> Divide4/2, Divide3/2, Divide2/2, Gain4/1
  Matrix Concatenate/1 -> coef_qdd/1
  Divide3/1 -> Matrix Concatenate/5
  Math Function4/1 -> Gain3/1
  Constant3/1 -> Math Function3/2
  Divide2/1 -> Matrix Concatenate/4
  Constant4/1 -> Math Function4/2
  Math Function3/1 -> Gain2/1
  t/1 -> Math Function3/1, Math Function4/1, Math Function2/1
  Constant2/1 -> Math Function2/2
  Math Function2/1 -> Gain1/1
  Divide4/1 -> Matrix Concatenate/6
  Gain4/1 -> Matrix Concatenate/3

== system animation/Trajectory Generator/Trajectory2/A ==
  Constant : Constant  Value=[eye(6) T*eye(6) T^2*eye(6) T^3*eye(6) T^4*eye(6) T^5*eye(6)]
  Constant1 : Constant  Value=[eye(6) 2*eye(6)*T 4*eye(6)*T^2 8*eye(6)*T^3 16*eye(6)*T^4 32*eye(6)*T^5]
  Constant2 : Constant  Value=[zeros(6) eye(6) eye(6)*2*T eye(6)*3*T^2 eye(6)*4*T^3 eye(6)*5*T^4]
  Constant3 : Constant  Value=[zeros(6) eye(6) eye(6)*4*T eye(6)*12*T^2 eye(6)*32*T^3 eye(6)*80*T^4]
  Constant4 : Constant  Value=[zeros(6) zeros(6) 2*eye(6) 6*T*eye(6) 12*T^2*eye(6) 20*T^3*eye(6)]
  Constant5 : Constant  Value=[zeros(6) zeros(6) 2*eye(6) 12*T*eye(6) 48*T^2*eye(6) 160*T^3*eye(6)]
  Divide : Product  Inputs=/  Multiplication=Matrix(*)
  Matrix Concatenate : Concatenate  NumInputs=6  Mode=Multidimensional array
  Matrix Concatenate1 : Concatenate  NumInputs=6  Mode=Multidimensional array
  O{1..4} (4 alike) : Constant  Value=zeros(6,1)
  Product : Product  Multiplication=Matrix(*)
  q_2T : Constant  Value=q2
  q_T : Constant  Value=q1
  A : Outport
  wires:
  Product/1 -> A/1
  Divide/1 -> Product/1
  Matrix Concatenate/1 -> Product/2
  Matrix Concatenate1/1 -> Divide/1
  Constant5/1 -> Matrix Concatenate1/6
  Constant4/1 -> Matrix Concatenate1/5
  Constant3/1 -> Matrix Concatenate1/4
  Constant2/1 -> Matrix Concatenate1/3
  Constant1/1 -> Matrix Concatenate1/2
  Constant/1 -> Matrix Concatenate1/1
  O1/1 -> Matrix Concatenate/3
  O2/1 -> Matrix Concatenate/4
  O4/1 -> Matrix Concatenate/6
  O3/1 -> Matrix Concatenate/5
  q_T/1 -> Matrix Concatenate/1
  q_2T/1 -> Matrix Concatenate/2

== system animation/Trajectory Generator/Trajectory2/coef_q ==
  t : Inport
  Constant1 : Constant  Value=2
  Constant2 : Constant  Value=3
  Constant3 : Constant  Value=4
  Constant4 : Constant  Value=5
  Divide{,1..4} (5 alike) : Product  Inputs=**
  I : Constant  Value=eye(6)
  Math Function{1..4} (4 alike) : Math  Operator=pow  SaturateOnIntegerOverflow=on
  Matrix Concatenate : Concatenate  NumInputs=6  Mode=Multidimensional array  ConcatenateDimension=2
  coef_q : Outport
  wires:
  Divide4/1 -> Matrix Concatenate/6
  Math Function2/1 -> Divide2/1
  Constant2/1 -> Math Function2/2
  Math Function1/1 -> Divide1/1
  t/1 -> Math Function1/1, Math Function2/1, Math Function4/1, Math Function3/1, Divide/1
  Math Function3/1 -> Divide3/1
  Constant4/1 -> Math Function4/2
  Divide2/1 -> Matrix Concatenate/4
  Constant3/1 -> Math Function3/2
  Math Function4/1 -> Divide4/1
  Divide1/1 -> Matrix Concatenate/3
  Divide3/1 -> Matrix Concatenate/5
  Constant1/1 -> Math Function1/2
  I/1 -> Divide/2, Divide1/2, Divide2/2, Divide3/2, Divide4/2, Matrix Concatenate/1
  Matrix Concatenate/1 -> coef_q/1
  Divide/1 -> Matrix Concatenate/2

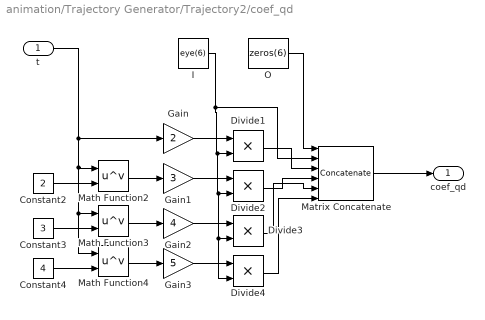
== system animation/Trajectory Generator/Trajectory2/coef_qd ==
  t : Inport
  Constant2 : Constant  Value=2
  Constant3 : Constant  Value=3
  Constant4 : Constant  Value=4
  Divide{1..4} (4 alike) : Product  Inputs=**
  Gain : Gain  Gain=2
  Gain1 : Gain  Gain=3
  Gain2 : Gain  Gain=4
  Gain3 : Gain  Gain=5
  I : Constant  Value=eye(6)
  Math Function2 : Math  Operator=pow  SaturateOnIntegerOverflow=on
  Math Function3 : Math  Operator=pow  SaturateOnIntegerOverflow=on
  Math Function4 : Math  Operator=pow  SaturateOnIntegerOverflow=on
  Matrix Concatenate : Concatenate  NumInputs=6  Mode=Multidimensional array  ConcatenateDimension=2
  O : Constant  Value=zeros(6)
  coef_qd : Outport
  wires:
  Gain3/1 -> Divide4/1
  Gain2/1 -> Divide3/1
  Gain1/1 -> Divide2/1
  Gain/1 -> Divide1/1
  O/1 -> Matrix Concatenate/1
  I/1 -> Divide4/2, Divide3/2, Divide2/2, Divide1/2, Matrix Concatenate/2
  Matrix Concatenate/1 -> coef_qd/1
  Divide3/1 -> Matrix Concatenate/5
  Divide1/1 -> Matrix Concatenate/3
  Math Function4/1 -> Gain3/1
  Constant3/1 -> Math Function3/2
  Divide2/1 -> Matrix Concatenate/4
  Constant4/1 -> Math Function4/2
  Math Function3/1 -> Gain2/1
  t/1 -> Math Function3/1, Math Function4/1, Math Function2/1, Gain/1
  Constant2/1 -> Math Function2/2
  Math Function2/1 -> Gain1/1
  Divide4/1 -> Matrix Concatenate/6

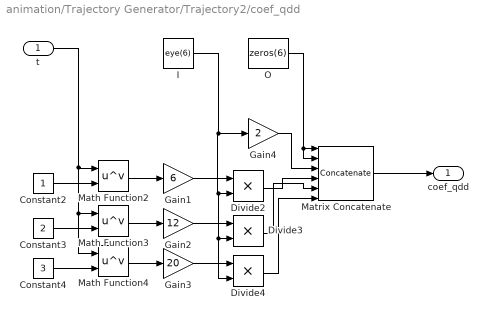
== system animation/Trajectory Generator/Trajectory2/coef_qdd ==
  t : Inport
  Constant2 : Constant
  Constant3 : Constant  Value=2
  Constant4 : Constant  Value=3
  Divide2 : Product  Inputs=**
  Divide3 : Product  Inputs=**
  Divide4 : Product  Inputs=**
  Gain1 : Gain  Gain=6
  Gain2 : Gain  Gain=12
  Gain3 : Gain  Gain=20
  Gain4 : Gain  Gain=2
  I : Constant  Value=eye(6)
  Math Function2 : Math  Operator=pow  SaturateOnIntegerOverflow=on
  Math Function3 : Math  Operator=pow  SaturateOnIntegerOverflow=on
  Math Function4 : Math  Operator=pow  SaturateOnIntegerOverflow=on
  Matrix Concatenate : Concatenate  NumInputs=6  Mode=Multidimensional array  ConcatenateDimension=2
  O : Constant  Value=zeros(6)
  coef_qdd : Outport
  wires:
  Gain4/1 -> Matrix Concatenate/3
  Divide4/1 -> Matrix Concatenate/6
  Math Function2/1 -> Gain1/1
  Constant2/1 -> Math Function2/2
  t/1 -> Math Function2/1, Math Function4/1, Math Function3/1
  Math Function3/1 -> Gain2/1
  Constant4/1 -> Math Function4/2
  Divide2/1 -> Matrix Concatenate/4
  Constant3/1 -> Math Function3/2
  Math Function4/1 -> Gain3/1
  Divide3/1 -> Matrix Concatenate/5
  Matrix Concatenate/1 -> coef_qdd/1
  I/1 -> Gain4/1, Divide2/2, Divide3/2, Divide4/2
  O/1 -> Matrix Concatenate/1, Matrix Concatenate/2
  Gain1/1 -> Divide2/1
  Gain2/1 -> Divide3/1
  Gain3/1 -> Divide4/1

== system animation/Trajectory Generator/Trajectory3/A ==
  Constant1 : Constant  Value=[eye(6) 2*eye(6)*T 4*eye(6)*T^2 8*eye(6)*T^3 16*eye(6)*T^4 32*eye(6)*T^5]
  Constant2 : Constant  Value=[zeros(6) eye(6) eye(6)*4*T eye(6)*12*T^2 eye(6)*32*T^3 eye(6)*80*T^4]
  Constant3 : Constant  Value=[zeros(6) eye(6) eye(6)*6*T eye(6)*27*T^2 eye(6)*108*T^3 eye(6)*405*T^4]
  Constant4 : Constant  Value=[zeros(6) zeros(6) 2*eye(6) 12*T*eye(6) 48*T^2*eye(6) 160*T^3*eye(6)]
  Constant5 : Constant  Value=[zeros(6) zeros(6) 2*eye(6) 18*T*eye(6) 108*T^2*eye(6) 540*T^3*eye(6)]
  Constant6 : Constant  Value=[eye(6) 3*eye(6)*T 9*eye(6)*T^2 27*eye(6)*T^3 81*eye(6)*T^4 243*eye(6)*T^5]
  Divide : Product  Inputs=/  Multiplication=Matrix(*)
  Matrix Concatenate : Concatenate  NumInputs=6  Mode=Multidimensional array
  Matrix Concatenate1 : Concatenate  NumInputs=6  Mode=Multidimensional array
  O{,1..4} (5 alike) : Constant  Value=zeros(6,1)
  Product : Product  Multiplication=Matrix(*)
  q_T : Constant  Value=q2
  A : Outport
  wires:
  O/1 -> Matrix Concatenate/2
  q_T/1 -> Matrix Concatenate/1
  O3/1 -> Matrix Concatenate/5
  O4/1 -> Matrix Concatenate/6
  O2/1 -> Matrix Concatenate/4
  O1/1 -> Matrix Concatenate/3
  Constant2/1 -> Matrix Concatenate1/3
  Constant4/1 -> Matrix Concatenate1/5
  Constant5/1 -> Matrix Concatenate1/6
  Matrix Concatenate1/1 -> Divide/1
  Matrix Concatenate/1 -> Product/2
  Divide/1 -> Product/1
  Product/1 -> A/1
  Constant1/1 -> Matrix Concatenate1/1
  Constant6/1 -> Matrix Concatenate1/2
  Constant3/1 -> Matrix Concatenate1/4

== system animation/Trajectory Generator/Trajectory3/coef_q ==
  t : Inport
  Constant1 : Constant  Value=2
  Constant2 : Constant  Value=3
  Constant3 : Constant  Value=4
  Constant4 : Constant  Value=5
  Divide{,1..4} (5 alike) : Product  Inputs=**
  I : Constant  Value=eye(6)
  Math Function{1..4} (4 alike) : Math  Operator=pow  SaturateOnIntegerOverflow=on
  Matrix Concatenate : Concatenate  NumInputs=6  Mode=Multidimensional array  ConcatenateDimension=2
  coef_q : Outport
  wires:
  Divide/1 -> Matrix Concatenate/2
  Matrix Concatenate/1 -> coef_q/1
  I/1 -> Matrix Concatenate/1, Divide4/2, Divide3/2, Divide2/2, Divide1/2, Divide/2
  Constant1/1 -> Math Function1/2
  Divide3/1 -> Matrix Concatenate/5
  Divide1/1 -> Matrix Concatenate/3
  Math Function4/1 -> Divide4/1
  Constant3/1 -> Math Function3/2
  Divide2/1 -> Matrix Concatenate/4
  Constant4/1 -> Math Function4/2
  Math Function3/1 -> Divide3/1
  t/1 -> Divide/1, Math Function3/1, Math Function4/1, Math Function2/1, Math Function1/1
  Math Function1/1 -> Divide1/1
  Constant2/1 -> Math Function2/2
  Math Function2/1 -> Divide2/1
  Divide4/1 -> Matrix Concatenate/6

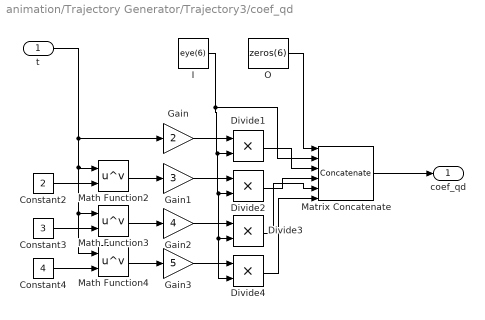
== system animation/Trajectory Generator/Trajectory3/coef_qd ==
  t : Inport
  Constant2 : Constant  Value=2
  Constant3 : Constant  Value=3
  Constant4 : Constant  Value=4
  Divide{1..4} (4 alike) : Product  Inputs=**
  Gain : Gain  Gain=2
  Gain1 : Gain  Gain=3
  Gain2 : Gain  Gain=4
  Gain3 : Gain  Gain=5
  I : Constant  Value=eye(6)
  Math Function2 : Math  Operator=pow  SaturateOnIntegerOverflow=on
  Math Function3 : Math  Operator=pow  SaturateOnIntegerOverflow=on
  Math Function4 : Math  Operator=pow  SaturateOnIntegerOverflow=on
  Matrix Concatenate : Concatenate  NumInputs=6  Mode=Multidimensional array  ConcatenateDimension=2
  O : Constant  Value=zeros(6)
  coef_qd : Outport
  wires:
  Divide4/1 -> Matrix Concatenate/6
  Math Function2/1 -> Gain1/1
  Constant2/1 -> Math Function2/2
  t/1 -> Gain/1, Math Function2/1, Math Function4/1, Math Function3/1
  Math Function3/1 -> Gain2/1
  Constant4/1 -> Math Function4/2
  Divide2/1 -> Matrix Concatenate/4
  Constant3/1 -> Math Function3/2
  Math Function4/1 -> Gain3/1
  Divide1/1 -> Matrix Concatenate/3
  Divide3/1 -> Matrix Concatenate/5
  Matrix Concatenate/1 -> coef_qd/1
  I/1 -> Matrix Concatenate/2, Divide1/2, Divide2/2, Divide3/2, Divide4/2
  O/1 -> Matrix Concatenate/1
  Gain/1 -> Divide1/1
  Gain1/1 -> Divide2/1
  Gain2/1 -> Divide3/1
  Gain3/1 -> Divide4/1

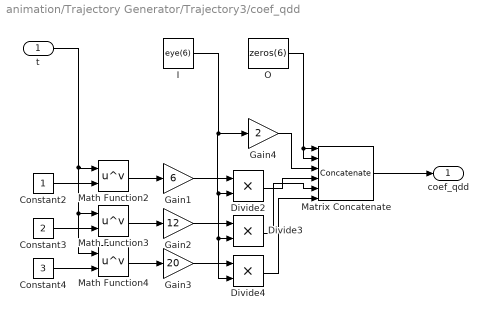
== system animation/Trajectory Generator/Trajectory3/coef_qdd ==
  t : Inport
  Constant2 : Constant
  Constant3 : Constant  Value=2
  Constant4 : Constant  Value=3
  Divide2 : Product  Inputs=**
  Divide3 : Product  Inputs=**
  Divide4 : Product  Inputs=**
  Gain1 : Gain  Gain=6
  Gain2 : Gain  Gain=12
  Gain3 : Gain  Gain=20
  Gain4 : Gain  Gain=2
  I : Constant  Value=eye(6)
  Math Function2 : Math  Operator=pow  SaturateOnIntegerOverflow=on
  Math Function3 : Math  Operator=pow  SaturateOnIntegerOverflow=on
  Math Function4 : Math  Operator=pow  SaturateOnIntegerOverflow=on
  Matrix Concatenate : Concatenate  NumInputs=6  Mode=Multidimensional array  ConcatenateDimension=2
  O : Constant  Value=zeros(6)
  coef_qdd : Outport
  wires:
  Gain3/1 -> Divide4/1
  Gain2/1 -> Divide3/1
  Gain1/1 -> Divide2/1
  O/1 -> Matrix Concatenate/2, Matrix Concatenate/1
  I/1 -> Divide4/2, Divide3/2, Divide2/2, Gain4/1
  Matrix Concatenate/1 -> coef_qdd/1
  Divide3/1 -> Matrix Concatenate/5
  Math Function4/1 -> Gain3/1
  Constant3/1 -> Math Function3/2
  Divide2/1 -> Matrix Concatenate/4
  Constant4/1 -> Math Function4/2
  Math Function3/1 -> Gain2/1
  t/1 -> Math Function3/1, Math Function4/1, Math Function2/1
  Constant2/1 -> Math Function2/2
  Math Function2/1 -> Gain1/1
  Divide4/1 -> Matrix Concatenate/6
  Gain4/1 -> Matrix Concatenate/3

== system animation/Trajectory Generator1/Trajectory2/A ==
  Constant : Constant  Value=[eye(6) zeros(6) zeros(6) zeros(6) zeros(6) zeros(6)]
  Constant1 : Constant  Value=[eye(6) eye(6)*T eye(6)*T^2 eye(6)*T^3 eye(6)*T^4 eye(6)*T^5]
  Constant2 : Constant  Value=[zeros(6) eye(6) zeros(6) zeros(6) zeros(6) zeros(6)]
  Constant3 : Constant  Value=[zeros(6) eye(6) eye(6)*2*T eye(6)*3*T^2 eye(6)*4*T^3 eye(6)*5*T^4]
  Constant4 : Constant  Value=[zeros(6) zeros(6) 2*eye(6) zeros(6) zeros(6) zeros(6)]
  Constant5 : Constant  Value=[zeros(6) zeros(6) 2*eye(6) 6*T*eye(6) 12*T^2*eye(6) 20*T^3*eye(6)]
  Divide : Product  Inputs=/  Multiplication=Matrix(*)
  Matrix Concatenate : Concatenate  NumInputs=6  Mode=Multidimensional array
  Matrix Concatenate1 : Concatenate  NumInputs=6  Mode=Multidimensional array
  O{,1..4} (5 alike) : Constant  Value=zeros(6,1)
  Product : Product  Multiplication=Matrix(*)
  q_T : Constant  Value=[q1;q2;q3;q4;q5;q6]
  A : Outport
  wires:
  O3/1 -> Matrix Concatenate/5
  O/1 -> Matrix Concatenate/1
  q_T/1 -> Matrix Concatenate/2
  O4/1 -> Matrix Concatenate/6
  O2/1 -> Matrix Concatenate/4
  O1/1 -> Matrix Concatenate/3
  Constant/1 -> Matrix Concatenate1/1
  Constant1/1 -> Matrix Concatenate1/2
  Constant2/1 -> Matrix Concatenate1/3
  Constant3/1 -> Matrix Concatenate1/4
  Constant4/1 -> Matrix Concatenate1/5
  Constant5/1 -> Matrix Concatenate1/6
  Matrix Concatenate1/1 -> Divide/1
  Matrix Concatenate/1 -> Product/2
  Divide/1 -> Product/1
  Product/1 -> A/1

== system animation/Trajectory Generator1/Trajectory2/coef_q ==
  t : Inport
  Constant1 : Constant  Value=2
  Constant2 : Constant  Value=3
  Constant3 : Constant  Value=4
  Constant4 : Constant  Value=5
  Divide{,1..4} (5 alike) : Product  Inputs=**
  I : Constant  Value=eye(6)
  Math Function{1..4} (4 alike) : Math  Operator=pow  SaturateOnIntegerOverflow=on
  Matrix Concatenate : Concatenate  NumInputs=6  Mode=Multidimensional array  ConcatenateDimension=2
  coef_q : Outport
  wires:
  Divide/1 -> Matrix Concatenate/2
  Matrix Concatenate/1 -> coef_q/1
  I/1 -> Matrix Concatenate/1, Divide4/2, Divide3/2, Divide2/2, Divide1/2, Divide/2
  Constant1/1 -> Math Function1/2
  Divide3/1 -> Matrix Concatenate/5
  Divide1/1 -> Matrix Concatenate/3
  Math Function4/1 -> Divide4/1
  Constant3/1 -> Math Function3/2
  Divide2/1 -> Matrix Concatenate/4
  Constant4/1 -> Math Function4/2
  Math Function3/1 -> Divide3/1
  t/1 -> Divide/1, Math Function3/1, Math Function4/1, Math Function2/1, Math Function1/1
  Math Function1/1 -> Divide1/1
  Constant2/1 -> Math Function2/2
  Math Function2/1 -> Divide2/1
  Divide4/1 -> Matrix Concatenate/6

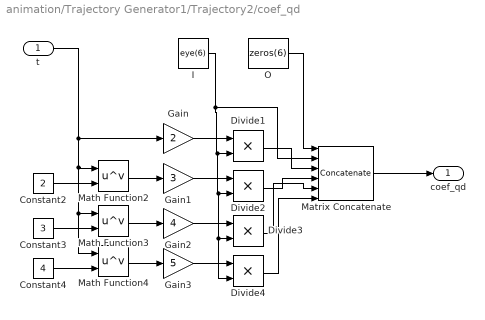
== system animation/Trajectory Generator1/Trajectory2/coef_qd ==
  t : Inport
  Constant2 : Constant  Value=2
  Constant3 : Constant  Value=3
  Constant4 : Constant  Value=4
  Divide{1..4} (4 alike) : Product  Inputs=**
  Gain : Gain  Gain=2
  Gain1 : Gain  Gain=3
  Gain2 : Gain  Gain=4
  Gain3 : Gain  Gain=5
  I : Constant  Value=eye(6)
  Math Function2 : Math  Operator=pow  SaturateOnIntegerOverflow=on
  Math Function3 : Math  Operator=pow  SaturateOnIntegerOverflow=on
  Math Function4 : Math  Operator=pow  SaturateOnIntegerOverflow=on
  Matrix Concatenate : Concatenate  NumInputs=6  Mode=Multidimensional array  ConcatenateDimension=2
  O : Constant  Value=zeros(6)
  coef_qd : Outport
  wires:
  Divide4/1 -> Matrix Concatenate/6
  Math Function2/1 -> Gain1/1
  Constant2/1 -> Math Function2/2
  t/1 -> Gain/1, Math Function2/1, Math Function4/1, Math Function3/1
  Math Function3/1 -> Gain2/1
  Constant4/1 -> Math Function4/2
  Divide2/1 -> Matrix Concatenate/4
  Constant3/1 -> Math Function3/2
  Math Function4/1 -> Gain3/1
  Divide1/1 -> Matrix Concatenate/3
  Divide3/1 -> Matrix Concatenate/5
  Matrix Concatenate/1 -> coef_qd/1
  I/1 -> Matrix Concatenate/2, Divide1/2, Divide2/2, Divide3/2, Divide4/2
  O/1 -> Matrix Concatenate/1
  Gain/1 -> Divide1/1
  Gain1/1 -> Divide2/1
  Gain2/1 -> Divide3/1
  Gain3/1 -> Divide4/1

== system animation/Trajectory Generator1/Trajectory2/coef_qdd ==
  t : Inport
  Constant2 : Constant
  Constant3 : Constant  Value=2
  Constant4 : Constant  Value=3
  Divide2 : Product  Inputs=**
  Divide3 : Product  Inputs=**
  Divide4 : Product  Inputs=**
  Gain1 : Gain  Gain=6
  Gain2 : Gain  Gain=12
  Gain3 : Gain  Gain=20
  Gain4 : Gain  Gain=2
  I : Constant  Value=eye(6)
  Math Function2 : Math  Operator=pow  SaturateOnIntegerOverflow=on
  Math Function3 : Math  Operator=pow  SaturateOnIntegerOverflow=on
  Math Function4 : Math  Operator=pow  SaturateOnIntegerOverflow=on
  Matrix Concatenate : Concatenate  NumInputs=6  Mode=Multidimensional array  ConcatenateDimension=2
  O : Constant  Value=zeros(6)
  coef_qdd : Outport
  wires:
  Gain3/1 -> Divide4/1
  Gain2/1 -> Divide3/1
  Gain1/1 -> Divide2/1
  O/1 -> Matrix Concatenate/2, Matrix Concatenate/1
  I/1 -> Divide4/2, Divide3/2, Divide2/2, Gain4/1
  Matrix Concatenate/1 -> coef_qdd/1
  Divide3/1 -> Matrix Concatenate/5
  Math Function4/1 -> Gain3/1
  Constant3/1 -> Math Function3/2
  Divide2/1 -> Matrix Concatenate/4
  Constant4/1 -> Math Function4/2
  Math Function3/1 -> Gain2/1
  t/1 -> Math Function3/1, Math Function4/1, Math Function2/1
  Constant2/1 -> Math Function2/2
  Math Function2/1 -> Gain1/1
  Divide4/1 -> Matrix Concatenate/6
  Gain4/1 -> Matrix Concatenate/3

== system animation/Control Policies/Inverse Dynamics Control/Inverse Dynamics/Link0 ==
  Rigid Transform : sm_lib/Frames and Transforms/Rigid Transform  TranslationMethod=None  TranslationStandardOffset=0  TranslationLengthUnit=m  TranslationStandardAxis=+Z  TranslationCartesianOffset=[0 0 0]  TranslationROffset=0  TranslationROffsetUnits=m  TranslationZOffset=0  TranslationZOffsetUnits=m  TranslationThetaOffset=0  TranslationThetaOffsetUnits=deg  RotationMethod=StandardAxis  RotationAngleUnits=rad  RotationStandardAxis=+Z  RotationAngle=pi  RotationArbitraryAxis=[0 0 1]  FollAlignAxisA=+X  BaseAlignAxisA=+Y  FollAlignAxisB=+Y  BaseAlignAxisB=+Z  RotationSequenceAxes=FollowerAxes  RotationSequence=XYX  RotationSequenceAngles=[0 0 0]  RotationSequenceAnglesUnits=deg  RotationMatrix=[1 0 0; 0 1 0; 0 0 1]
  Solid : sm_lib/Body Elements/Solid  InertiaType=Custom  Mass=12.21  MassUnits=kg  CenterOfMass=[53.3 2.09 37.75]  CenterOfMassUnits=mm  MomentsOfInertia=[0.27 0.33 0.54]  MomentsOfInertiaUnits=kg*m^2  ProductsOfInertia=[0 0.03 0.01]  ProductsOfInertiaUnits=kg*m^2  BasedOnType=Density  Density=1000  DensityUnits=kg/m^3  DoExposeReferenceFrame=on  SerializedFrames=<Frames/>  GraphicType=FromGeometry  MarkerShape=Sphere  MarkerSize=10  GraphicVisPropType=SimpleVisualProperties  GraphicDiffuseColor=[0.5 0.5 0.5]  GraphicSpecularColor=[0.5 0.5 0.5 1.0]  GraphicAmbientColor=[0.15 0.15 0.15 1.0]  GraphicEmissiveColor=[0.0 0.0 0.0 1.0]  GraphicShininess=75  GraphicOpacity=1.0  GeometryShape=FromFile  RectangleSize=[1 1]  RectangleSizeUnits=m  BrickDimensions=[1 1 1]  BrickDimensionUnits=m  CylinderRadius=1  CylinderRadiusUnits=m  CylinderLength=1  CylinderLengthUnits=m  SphereRadius=1  SphereRadiusUnits=m  EllipsoidRadii=[1 1 1]  EllipsoidRadiiUnits=m  ExtrusionCrossSection=[1 1; -1 1; -1 -1; 1 -1]  ExtrusionCrossSectionUnits=m  ExtrusionLength=1  ExtrusionLengthUnits=m  PolygonNumSides=3  PolygonOuterRadius=1  PolygonOuterRadiusUnits=m  ExtGeomFileType=STL  ExtGeomFileName=D:\Chin\3rdYearsProject\IntroRobotics\Project\CAD\Assem0+frame.STL  ExtGeomFileUnits=mm  RevolutionCrossSection=[1 1; 1 -1; 2 -1; 2 1]  RevolutionCrossSectionUnits=m  RevolutionExtent=Full  RevolutionAngle=180  RevolutionAngleUnits=deg
  Frame0 : PMIOPort  Side=Left
  World Frame : PMIOPort  Port=2  Side=Left
  connections:
  World Frame/RConn1 -- Rigid Transform/LConn1
  Frame0/RConn1 -- Solid/RConn1 -- Rigid Transform/RConn1
